simulink model "hand_simulator_v4"  (R2023b)
settings: Solver=VariableStepAuto  StartTime=0.0  StopTime=0  FixedStep=1e-2  RelTol=1e-3
PreLoadFcn:
  | addpath("functions\HandModel\HumanHand\")
undefined symbols (not defined in the file): ts, X, Y, Z
libraries: sm_lib x211, nesl_utility x56
(part 1 of 6)
settings Model: Creator=chopp  LastModifiedBy=chopp
settings ExplorerConfigSet: InternalSimMechanicsExplorerSettings="<ExplorerConfiguration><canonicalview>default</canonicalview><AnimationSetting><BasePlaybackSpeed>1.0</BasePlaybackSpeed><PlaybackSpeedFactor>1.0</PlaybackSpeedFactor></AnimationSetting><TilePanel><TileInfo><Tiles Columns=\"1\" Count=\"1\" Rows=\"1\"><Column Weight=\"1\"/><Row Weight=\"1\"/><Tile Height=\"1\" Width=\"1\" X=\"0\" Y=\"0\"/></Tiles></TileInfo><SceneInfo><SceneViewer><BGColor><R>1</R><G>1</G><B>1</B></BGColor><Camera><DoPerspective>on</DoPerspective><Position><X>0.119329689227050506</X><Y>0.117433489686037784</Y><Z>0.124504754223393604</Z></Position><Center><X>0.0300118695298526722</X><Y>0.0234238145278355299</Y><Z>0.0378621546990252772</Z></Center><Up><X>0.816868216190496765</X><Y>-0.362790797954974598</Y><Z>-0.448451953164381412</Z></Up><ViewLimDist>1</ViewLimDist><YLim>0.466307658154998583</YLim><XLim>0.634472152198297223</XLim></Camera></SceneViewer></SceneInfo></TilePanel><MechEditorPanel><Cameras><Camera><Id>Camera1</Id><Value><Name>Camera1</Name><NativeCamera><PositionKeyframeSet><Keyframe><Time>0</Time><Value><X>0.11932968922705051</X><Y>0.11743348968603778</Y><Z>0.1245047542233936</Z></Value></Keyframe></PositionKeyframeSet><CenterKeyframeSet><Keyframe><Time>0</Time><Value><X>0.030011869529852672</X><Y>0.02342381452783553</Y><Z>0.037862154699025277</Z></Value></Keyframe></CenterKeyframeSet><UpVectorKeyframeSet><Keyframe><Time>0</Time><Value><X>0.81686821619049677</X><Y>-0.3627907979549746</Y><Z>-0.44845195316438141</Z></Value></Keyframe></UpVectorKeyframeSet></NativeCamera></Value></Camera></Cameras><GfxPanelCameraMap><MapElement CameraMLId=\"Camera1\" GfxPanelIndex=\"0\"/></GfxPanelCameraMap><VideoCreator><PlaybackSpeedRatio>1.0</PlaybackSpeedRatio><FrameRate>30</FrameRate><VideoFormat>Motion JPEG AVI</VideoFormat><FrameSize>auto</FrameSize></VideoCreator></MechEditorPanel></ExplorerConfiguration>"

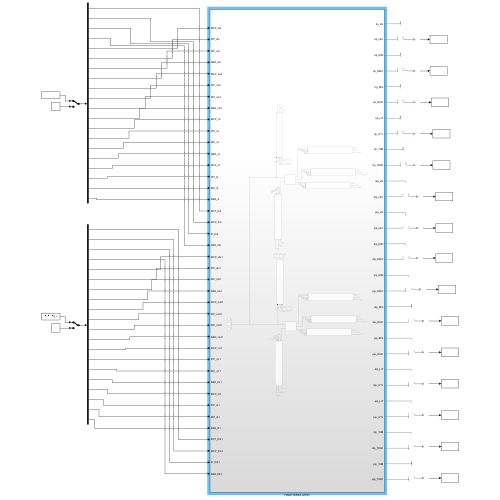
[thumbnail: Simulink's stored preview of the top-level diagram]
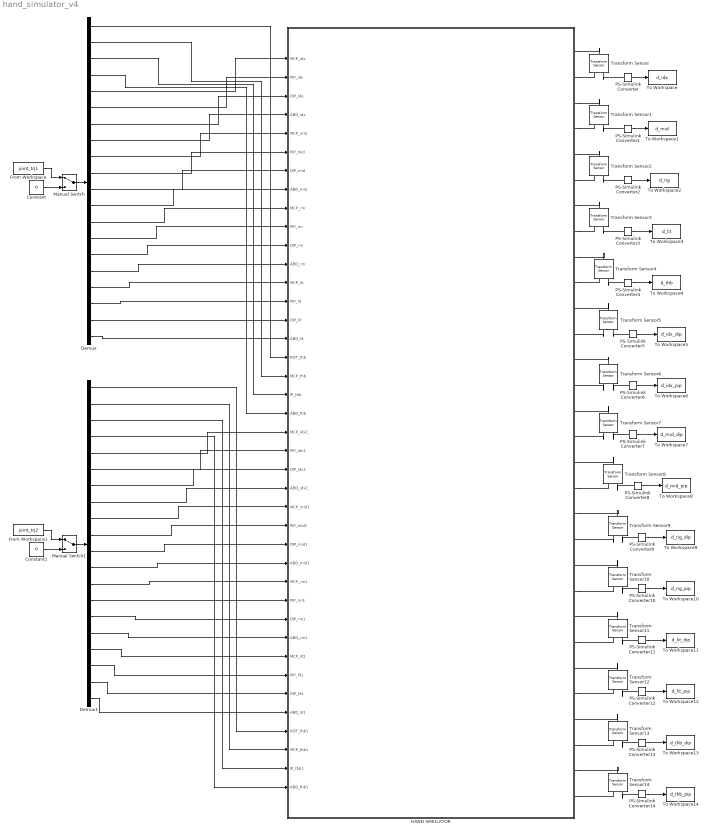
== system hand_simulator_v4 ==
  Constant : Constant  Value=0
  Constant1 : Constant  Value=0
  Demux : Demux  Outputs=20
  Demux1 : Demux  Outputs=20
  From Workspace : FromWorkspace  VariableName=joint_trj1  SampleTime=ts
  From Workspace1 : FromWorkspace  VariableName=joint_trj2  SampleTime=ts
  HAND SIMULATOR : Subsystem
  Manual Switch : ManualSwitch
  Manual Switch1 : ManualSwitch
  PS-Simulink Converter{,1..14} (15 alike) : nesl_utility/PS-Simulink Converter  PhysicalDomain=network_engine_domain  SubClassName=ps_output  LeftPortType=input  RightPortType=output  PseudoPeriodic=off  Frequencies=[]  VectorFormat=inherit  Unit=m  AffineConversion=off
  To Workspace : ToWorkspace  VariableName=d_idx  SaveFormat=Timeseries  SampleTime=0.01
  To Workspace1 : ToWorkspace  VariableName=d_mid  SaveFormat=Timeseries  SampleTime=0.01
  To Workspace10 : ToWorkspace  VariableName=d_rig_pip  SaveFormat=Timeseries  SampleTime=0.01
  To Workspace11 : ToWorkspace  VariableName=d_lit_dip  SaveFormat=Timeseries  SampleTime=0.01
  To Workspace12 : ToWorkspace  VariableName=d_lit_pip  SaveFormat=Timeseries  SampleTime=0.01
  To Workspace13 : ToWorkspace  VariableName=d_thb_dip  SaveFormat=Timeseries  SampleTime=0.01
  To Workspace14 : ToWorkspace  VariableName=d_thb_pip  SaveFormat=Timeseries  SampleTime=0.01
  To Workspace2 : ToWorkspace  VariableName=d_rig  SaveFormat=Timeseries  SampleTime=0.01
  To Workspace3 : ToWorkspace  VariableName=d_lit  SaveFormat=Timeseries  SampleTime=0.01
  To Workspace4 : ToWorkspace  VariableName=d_thb  SaveFormat=Timeseries  SampleTime=0.01
  To Workspace5 : ToWorkspace  VariableName=d_idx_dip  SaveFormat=Timeseries  SampleTime=0.01
  To Workspace6 : ToWorkspace  VariableName=d_idx_pip  SaveFormat=Timeseries  SampleTime=0.01
  To Workspace7 : ToWorkspace  VariableName=d_mid_dip  SaveFormat=Timeseries  SampleTime=0.01
  To Workspace8 : ToWorkspace  VariableName=d_mid_pip  SaveFormat=Timeseries  SampleTime=0.01
  To Workspace9 : ToWorkspace  VariableName=d_rig_dip  SaveFormat=Timeseries  SampleTime=0.01
  Transform Sensor{,1..14} (15 alike) : sm_lib/Frames and Transforms/Transform Sensor  MeasurementFrame=World  RotationSequence=XYX  SenseAngle=off  SenseAxis=off  SenseQ=off  SenseR=off  SenseRotationSequence=off  SenseOmegaX=off  SenseOmegaY=off  SenseOmegaZ=off  SenseOmega=off  SenseQDot=off  SenseRDot=off  SenseRotationSequenceDot=off  SenseAlphaX=off  SenseAlphaY=off  SenseAlphaZ=off  SenseAlpha=off  SenseQDDot=off  SenseRDDot=off  SenseX=off  SenseY=off  SenseZ=off  SenseXYZ=off  SenseRad=off  SenseAzim=off  SenseDist=on  SenseInc=off  SenseXDot=off  SenseYDot=off  SenseZDot=off  SenseXYZDot=off  SenseRadDot=off  SenseAzimDot=off  SenseDistDot=off  SenseIncDot=off  SenseXDDot=off  SenseYDDot=off  SenseZDDot=off  SenseXYZDDot=off  SenseRadDDot=off  SenseAzimDDot=off  SenseDistDDot=off  SenseIncDDot=off
  wires:
  Manual Switch1/1 -> Demux1/1
  Demux1/20 -> HAND SIMULATOR/36(ABD_lit1)
  Manual Switch/1 -> Demux/1
  Demux1/12 -> HAND SIMULATOR/28(ABD_mid1)
  From Workspace/1 -> Manual Switch/1
  Demux/14 -> HAND SIMULATOR/10(PIP_rin)
  Demux/2 -> HAND SIMULATOR/18(MCP_thb)
  Demux1/2 -> HAND SIMULATOR/38(MCP_thb1)
  Demux/17 -> HAND SIMULATOR/13(MCP_lit)
  Constant1/1 -> Manual Switch1/2
  Constant/1 -> Manual Switch/2
  Demux/1 -> HAND SIMULATOR/17(ROT_thb)
  From Workspace1/1 -> Manual Switch1/1
  Demux/18 -> HAND SIMULATOR/14(PIP_lit)
  Demux/3 -> HAND SIMULATOR/19(IP_thb)
  Demux/4 -> HAND SIMULATOR/20(ABD_thb)
  PS-Simulink Converter1/1 -> To Workspace1/1
  Demux/5 -> HAND SIMULATOR/1(MCP_idx)
  Demux/16 -> HAND SIMULATOR/12(ABD_rin)
  Demux/6 -> HAND SIMULATOR/2(PIP_idx)
  Demux/7 -> HAND SIMULATOR/3(DIP_idx)
  Demux/8 -> HAND SIMULATOR/4(ABD_idx)
  Demux/9 -> HAND SIMULATOR/5(MCP_mid)
  Demux/20 -> HAND SIMULATOR/16(ABD_lit)
  Demux/10 -> HAND SIMULATOR/6(PIP_mid)
  Demux/11 -> HAND SIMULATOR/7(DIP_mid)
  Demux/12 -> HAND SIMULATOR/8(ABD_mid)
  Demux/13 -> HAND SIMULATOR/9(MCP_rin)
  Demux/15 -> HAND SIMULATOR/11(DIP_rin)
  Demux1/17 -> HAND SIMULATOR/33(MCP_lit1)
  Demux/19 -> HAND SIMULATOR/15(DIP_lit)
  Demux1/4 -> HAND SIMULATOR/40(ABD_thb1)
  Demux1/1 -> HAND SIMULATOR/37(ROT_thb1)
  Demux1/19 -> HAND SIMULATOR/35(DIP_lit1)
  Demux1/8 -> HAND SIMULATOR/24(ABD_idx1)
  Demux1/3 -> HAND SIMULATOR/39(IP_thb1)
  Demux1/5 -> HAND SIMULATOR/21(MCP_idx1)
  Demux1/6 -> HAND SIMULATOR/22(PIP_idx1)
  Demux1/7 -> HAND SIMULATOR/23(DIP_idx1)
  Demux1/9 -> HAND SIMULATOR/25(MCP_mid1)
  Demux1/10 -> HAND SIMULATOR/26(PIP_mid1)
  Demux1/11 -> HAND SIMULATOR/27(DIP_mid1)
  Demux1/13 -> HAND SIMULATOR/29(MCP_rin1)
  Demux1/14 -> HAND SIMULATOR/30(PIP_rin1)
  Demux1/15 -> HAND SIMULATOR/31(DIP_rin1)
  Demux1/16 -> HAND SIMULATOR/32(ABD_rin1)
  Demux1/18 -> HAND SIMULATOR/34(PIP_lit1)
  PS-Simulink Converter/1 -> To Workspace/1
  PS-Simulink Converter2/1 -> To Workspace2/1
  PS-Simulink Converter3/1 -> To Workspace3/1
  PS-Simulink Converter4/1 -> To Workspace4/1
  PS-Simulink Converter5/1 -> To Workspace5/1
  PS-Simulink Converter6/1 -> To Workspace6/1
  PS-Simulink Converter7/1 -> To Workspace7/1
  PS-Simulink Converter8/1 -> To Workspace8/1
  PS-Simulink Converter9/1 -> To Workspace9/1
  PS-Simulink Converter10/1 -> To Workspace10/1
  PS-Simulink Converter11/1 -> To Workspace11/1
  PS-Simulink Converter12/1 -> To Workspace12/1
  PS-Simulink Converter13/1 -> To Workspace13/1
  PS-Simulink Converter14/1 -> To Workspace14/1
  connections:
  Transform Sensor3/RConn2 -- PS-Simulink Converter3/LConn1
  HAND SIMULATOR/RConn5 -- Transform Sensor2/LConn1
  HAND SIMULATOR/RConn8 -- Transform Sensor3/RConn1
  HAND SIMULATOR/RConn9 -- Transform Sensor4/LConn1
  Transform Sensor1/RConn2 -- PS-Simulink Converter1/LConn1
  Transform Sensor2/RConn2 -- PS-Simulink Converter2/LConn1
  HAND SIMULATOR/RConn3 -- Transform Sensor1/LConn1
  Transform Sensor4/RConn2 -- PS-Simulink Converter4/LConn1
  HAND SIMULATOR/RConn6 -- Transform Sensor2/RConn1
  HAND SIMULATOR/RConn7 -- Transform Sensor3/LConn1
  HAND SIMULATOR/RConn1 -- Transform Sensor/LConn1
  HAND SIMULATOR/RConn2 -- Transform Sensor/RConn1
  HAND SIMULATOR/RConn4 -- Transform Sensor1/RConn1
  HAND SIMULATOR/RConn10 -- Transform Sensor4/RConn1
  Transform Sensor/RConn2 -- PS-Simulink Converter/LConn1
  Transform Sensor5/RConn1 -- HAND SIMULATOR/RConn12
  Transform Sensor5/RConn2 -- PS-Simulink Converter5/LConn1
  Transform Sensor5/LConn1 -- HAND SIMULATOR/RConn11
  Transform Sensor6/RConn2 -- PS-Simulink Converter6/LConn1
  Transform Sensor6/LConn1 -- HAND SIMULATOR/RConn13
  Transform Sensor6/RConn1 -- HAND SIMULATOR/RConn14
  Transform Sensor7/RConn1 -- HAND SIMULATOR/RConn16
  Transform Sensor7/LConn1 -- HAND SIMULATOR/RConn15
  Transform Sensor7/RConn2 -- PS-Simulink Converter7/LConn1
  Transform Sensor8/RConn2 -- PS-Simulink Converter8/LConn1
  HAND SIMULATOR/RConn18 -- Transform Sensor8/RConn1
  Transform Sensor8/LConn1 -- HAND SIMULATOR/RConn17
  Transform Sensor9/RConn2 -- PS-Simulink Converter9/LConn1
  Transform Sensor9/RConn1 -- HAND SIMULATOR/RConn20
  HAND SIMULATOR/RConn19 -- Transform Sensor9/LConn1
  Transform Sensor10/RConn2 -- PS-Simulink Converter10/LConn1
  HAND SIMULATOR/RConn22 -- Transform Sensor10/RConn1
  Transform Sensor10/LConn1 -- HAND SIMULATOR/RConn21
  Transform Sensor11/RConn2 -- PS-Simulink Converter11/LConn1
  HAND SIMULATOR/RConn24 -- Transform Sensor11/RConn1
  Transform Sensor11/LConn1 -- HAND SIMULATOR/RConn23
  Transform Sensor12/RConn2 -- PS-Simulink Converter12/LConn1
  HAND SIMULATOR/RConn26 -- Transform Sensor12/RConn1
  Transform Sensor12/LConn1 -- HAND SIMULATOR/RConn25
  Transform Sensor13/RConn2 -- PS-Simulink Converter13/LConn1
  HAND SIMULATOR/RConn28 -- Transform Sensor13/RConn1
  Transform Sensor13/LConn1 -- HAND SIMULATOR/RConn27
  Transform Sensor14/RConn2 -- PS-Simulink Converter14/LConn1
  HAND SIMULATOR/RConn30 -- Transform Sensor14/RConn1
  HAND SIMULATOR/RConn29 -- Transform Sensor14/LConn1

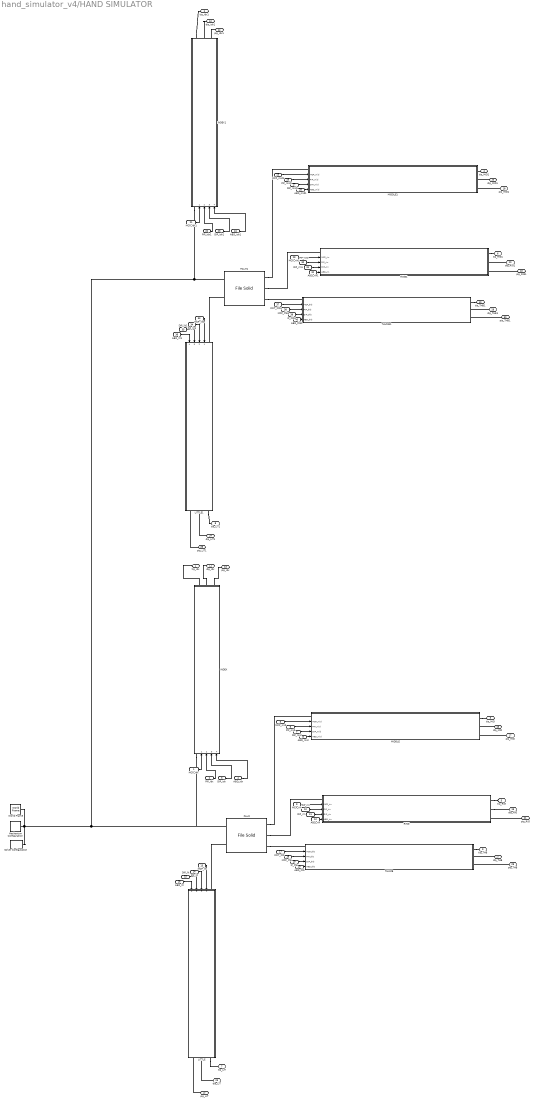
== system hand_simulator_v4/HAND SIMULATOR ==
  MCP_idx : Inport
  PIP_idx : Inport  Port=2
  DIP_idx : Inport  Port=3
  ABD_idx : Inport  Port=4
  MCP_mid : Inport  Port=5
  PIP_mid : Inport  Port=6
  DIP_mid : Inport  Port=7
  ABD_mid : Inport  Port=8
  MCP_rin : Inport  Port=9
  PIP_rin : Inport  Port=10
  DIP_rin : Inport  Port=11
  ABD_rin : Inport  Port=12
  MCP_lit : Inport  Port=13
  PIP_lit : Inport  Port=14
  DIP_lit : Inport  Port=15
  ABD_lit : Inport  Port=16
  ROT_thb : Inport  Port=17
  MCP_thb : Inport  Port=18
  IP_thb : Inport  Port=19
  ABD_thb : Inport  Port=20
  MCP_idx1 : Inport  Port=21
  PIP_idx1 : Inport  Port=22
  DIP_idx1 : Inport  Port=23
  ABD_idx1 : Inport  Port=24
  MCP_mid1 : Inport  Port=25
  PIP_mid1 : Inport  Port=26
  DIP_mid1 : Inport  Port=27
  ABD_mid1 : Inport  Port=28
  MCP_rin1 : Inport  Port=29
  PIP_rin1 : Inport  Port=30
  DIP_rin1 : Inport  Port=31
  ABD_rin1 : Inport  Port=32
  MCP_lit1 : Inport  Port=33
  PIP_lit1 : Inport  Port=34
  DIP_lit1 : Inport  Port=35
  ABD_lit1 : Inport  Port=36
  ROT_thb1 : Inport  Port=37
  MCP_thb1 : Inport  Port=38
  IP_thb1 : Inport  Port=39
  ABD_thb1 : Inport  Port=40
  INDEX : Subsystem
      settings: PortSchema="{\"entries\":[{\"content\":{\"sides\":[{\"content\":{\"connectorIds\":[\"LConn1\",\"In1\",\"In2\",\"In3\",\"In4\"]},\"type\":\"ConnectorPlacement.EquallySpacedRectSide\",\"uuid\":\"ba2071f2-d0ca-4999-8d8c-ca74a0e8f886\"},{\"content\":{\"connectorIds\":[\"RConn1\",\"RConn2\",\"RConn3\"],\"side\":\"RIGHT\"},\"type\":\"ConnectorPlacement.EquallySpacedRectSide\",\"uuid\":\"4961bf0d-9a2d-4923-b4f3-2392b2830b72\"},{\"content\":{\"side\":\"TOP\"},\"type\":\"ConnectorPlacement.EquallySpacedRectSide\",\"uuid\":\"0e6def02-82ab-4410-9cb6-5cc33d72600d\"}]},\"type\":\"ConnectorPlacement.EquallySpacedConnector\",\"uuid\":\"0dbe5955-5a93-4a14-ac05-25d414210df3\"}],\"packageUris\":[\"http://schema.mathworks.com/mf0/Connector/R2020b\"],\"version\":\"1.0\"}"
  INDEX1 : Subsystem
      settings: PortSchema="{\"entries\":[{\"content\":{\"sides\":[{\"content\":{\"connectorIds\":[\"LConn1\",\"In1\",\"In2\",\"In3\",\"In4\"]},\"type\":\"ConnectorPlacement.EquallySpacedRectSide\",\"uuid\":\"ba2071f2-d0ca-4999-8d8c-ca74a0e8f886\"},{\"content\":{\"connectorIds\":[\"RConn1\",\"RConn2\",\"RConn3\"],\"side\":\"RIGHT\"},\"type\":\"ConnectorPlacement.EquallySpacedRectSide\",\"uuid\":\"4961bf0d-9a2d-4923-b4f3-2392b2830b72\"},{\"content\":{\"side\":\"TOP\"},\"type\":\"ConnectorPlacement.EquallySpacedRectSide\",\"uuid\":\"0e6def02-82ab-4410-9cb6-5cc33d72600d\"}]},\"type\":\"ConnectorPlacement.EquallySpacedConnector\",\"uuid\":\"0dbe5955-5a93-4a14-ac05-25d414210df3\"}],\"packageUris\":[\"http://schema.mathworks.com/mf0/Connector/R2020b\"],\"version\":\"1.0\"}"
  LITTLE : Subsystem
      settings: PortSchema="{\"entries\":[{\"content\":{\"sides\":[{\"content\":{\"connectorIds\":[\"LConn1\",\"In1\",\"In2\",\"In3\",\"In4\"]},\"type\":\"ConnectorPlacement.EquallySpacedRectSide\",\"uuid\":\"6da030c9-b445-421e-a3aa-5870985b44ef\"},{\"content\":{\"connectorIds\":[\"RConn1\",\"RConn2\",\"RConn3\"],\"side\":\"RIGHT\"},\"type\":\"ConnectorPlacement.EquallySpacedRectSide\",\"uuid\":\"ddd1b4ad-e82e-4076-8ea7-1e0a4f531141\"},{\"content\":{\"side\":\"TOP\"},\"type\":\"ConnectorPlacement.EquallySpacedRectSide\",\"uuid\":\"430d8793-e7d8-4c1f-b03b-bab4880931cf\"}]},\"type\":\"ConnectorPlacement.EquallySpacedConnector\",\"uuid\":\"9c5926f4-db03-4b4c-81de-0122835d2650\"}],\"packageUris\":[\"http://schema.mathworks.com/mf0/Connector/R2020b\"],\"version\":\"1.0\"}"
  LITTLE1 : Subsystem
      settings: PortSchema="{\"entries\":[{\"content\":{\"sides\":[{\"content\":{\"connectorIds\":[\"LConn1\",\"In1\",\"In2\",\"In3\",\"In4\"]},\"type\":\"ConnectorPlacement.EquallySpacedRectSide\",\"uuid\":\"6da030c9-b445-421e-a3aa-5870985b44ef\"},{\"content\":{\"connectorIds\":[\"RConn1\",\"RConn2\",\"RConn3\"],\"side\":\"RIGHT\"},\"type\":\"ConnectorPlacement.EquallySpacedRectSide\",\"uuid\":\"ddd1b4ad-e82e-4076-8ea7-1e0a4f531141\"},{\"content\":{\"side\":\"TOP\"},\"type\":\"ConnectorPlacement.EquallySpacedRectSide\",\"uuid\":\"430d8793-e7d8-4c1f-b03b-bab4880931cf\"}]},\"type\":\"ConnectorPlacement.EquallySpacedConnector\",\"uuid\":\"9c5926f4-db03-4b4c-81de-0122835d2650\"}],\"packageUris\":[\"http://schema.mathworks.com/mf0/Connector/R2020b\"],\"version\":\"1.0\"}"
  MIDDLE : Subsystem
      settings: PortSchema="{\"entries\":[{\"content\":{\"sides\":[{\"content\":{\"connectorIds\":[\"LConn1\",\"In1\",\"In2\",\"In3\",\"In4\"]},\"type\":\"ConnectorPlacement.EquallySpacedRectSide\",\"uuid\":\"6da030c9-b445-421e-a3aa-5870985b44ef\"},{\"content\":{\"connectorIds\":[\"RConn1\",\"RConn2\",\"RConn3\"],\"side\":\"RIGHT\"},\"type\":\"ConnectorPlacement.EquallySpacedRectSide\",\"uuid\":\"ddd1b4ad-e82e-4076-8ea7-1e0a4f531141\"},{\"content\":{\"side\":\"TOP\"},\"type\":\"ConnectorPlacement.EquallySpacedRectSide\",\"uuid\":\"430d8793-e7d8-4c1f-b03b-bab4880931cf\"}]},\"type\":\"ConnectorPlacement.EquallySpacedConnector\",\"uuid\":\"9c5926f4-db03-4b4c-81de-0122835d2650\"}],\"packageUris\":[\"http://schema.mathworks.com/mf0/Connector/R2020b\"],\"version\":\"1.0\"}"
  MIDDLE1 : Subsystem
      settings: PortSchema="{\"entries\":[{\"content\":{\"sides\":[{\"content\":{\"connectorIds\":[\"LConn1\",\"In1\",\"In2\",\"In3\",\"In4\"]},\"type\":\"ConnectorPlacement.EquallySpacedRectSide\",\"uuid\":\"6da030c9-b445-421e-a3aa-5870985b44ef\"},{\"content\":{\"connectorIds\":[\"RConn1\",\"RConn2\",\"RConn3\"],\"side\":\"RIGHT\"},\"type\":\"ConnectorPlacement.EquallySpacedRectSide\",\"uuid\":\"ddd1b4ad-e82e-4076-8ea7-1e0a4f531141\"},{\"content\":{\"side\":\"TOP\"},\"type\":\"ConnectorPlacement.EquallySpacedRectSide\",\"uuid\":\"430d8793-e7d8-4c1f-b03b-bab4880931cf\"}]},\"type\":\"ConnectorPlacement.EquallySpacedConnector\",\"uuid\":\"9c5926f4-db03-4b4c-81de-0122835d2650\"}],\"packageUris\":[\"http://schema.mathworks.com/mf0/Connector/R2020b\"],\"version\":\"1.0\"}"
  Mechanism Configuration : sm_lib/Utilities/Mechanism Configuration  UniformGravity=Constant  GravityVector=[0 0 0]  GravityVectorUnits=m/s^2  LinearizationDelta=0.001  JointModeTransitionNonlinearIterations=2
  PALM : sm_lib/Body Elements/File Solid  ExtGeomFileName=palm.STEP  UnitType=FromFile  ExtGeomFileUnits=m  StepReaderType=HEX  ExportConvexHullGeometry=off  InertiaType=CalculateFromGeometry  Mass=1  MassUnits=kg  CenterOfMass=[0 0 0]  CenterOfMassUnits=m  MomentsOfInertia=[1 1 1]  MomentsOfInertiaUnits=kg*m^2  ProductsOfInertia=[0 0 0]  ProductsOfInertiaUnits=kg*m^2  BasedOnType=Density  Density=1000  DensityUnits=kg/m^3  DoExposeReferenceFrame=on  SerializedFrames=<Frames><Frame><Id>Frame1</Id><Value><Name>MID</Name><Origin><Source>GeometricFeature</Source><FeatureName>circular curve 11</FeatureName></Origin><PrimaryAxis><DefinedDirection>+Z</DefinedDirection><Source>ReferenceFrame</Source><SourceDirection>+Z</SourceDirection><FeatureName></FeatureName></PrimaryAxis><SecondaryAxis><DefinedDirection>+X</DefinedDirection><Source>ReferenceFrame</Source><SourceDirection>+X</SourceDirection><FeatureName></FeatureName></SecondaryAxis></Value></Frame><Frame><Id>Frame2</Id><Value><Name>RIG</Name><Origin><Source>GeometricFeature</Source><FeatureName>circular curve 6</FeatureName></Origin><PrimaryAxis><DefinedDirection>+Z</DefinedDirection><Source>ReferenceFrame</Source><SourceDirection>+Z</SourceDirection><FeatureName></FeatureName></PrimaryAxis><SecondaryAxis><DefinedDirection>+X</DefinedDirection><Source>ReferenceFrame</Source><SourceDirection>+X</SourceDirection><FeatureName></FeatureName></SecondaryAxis></Value></Frame><Frame><Id>Frame3</Id><Value><Name>LIT</Name><Origin><Source>GeometricFeature</Source><FeatureName>circular curve 2</FeatureName></Origin><PrimaryAxis><DefinedDirection>+Z</DefinedDirection><Source>ReferenceFrame</Source><SourceDirection>+Z</SourceDirection><FeatureName></FeatureName></PrimaryAxis><SecondaryAxis><DefinedDirection>+X</DefinedDirection><Source>ReferenceFrame</Source><SourceDirection>+X</SourceDirection><FeatureName></FeatureName></SecondaryAxis></Value></Frame><Frame><Id>Frame4</Id><Value><Name>THB</Name><Origin><Source>GeometricFeature</Source><FeatureName>circular curve 22</FeatureName></Origin><PrimaryAxis><DefinedDirection>+X</DefinedDirection><Source>ReferenceFrame</Source><SourceDirection>+Z</SourceDirection><FeatureName></FeatureName></PrimaryAxis><SecondaryAxis><DefinedDirection>+Y</DefinedDirection><Source>ReferenceFrame</Source><SourceDirection>+X</SourceDirection><FeatureName></FeatureName></SecondaryAxis></Value></Frame></Frames>  GraphicType=FromGeometry  MarkerShape=Sphere  MarkerSize=10  GraphicVisPropType=SimpleVisualProperties  GraphicDiffuseColor=[0.5 0.5 0.5]  GraphicSpecularColor=[0.5 0.5 0.5 1.0]  GraphicAmbientColor=[0.15 0.15 0.15 1.0]  GraphicEmissiveColor=[0.0 0.0 0.0 1.0]  GraphicShininess=75  GraphicOpacity=1.0
  PALM1 : sm_lib/Body Elements/File Solid  ExtGeomFileName=palm.STEP  UnitType=FromFile  ExtGeomFileUnits=m  StepReaderType=HEX  ExportConvexHullGeometry=off  InertiaType=CalculateFromGeometry  Mass=1  MassUnits=kg  CenterOfMass=[0 0 0]  CenterOfMassUnits=m  MomentsOfInertia=[1 1 1]  MomentsOfInertiaUnits=kg*m^2  ProductsOfInertia=[0 0 0]  ProductsOfInertiaUnits=kg*m^2  BasedOnType=Density  Density=1000  DensityUnits=kg/m^3  DoExposeReferenceFrame=on  SerializedFrames=<Frames><Frame><Id>Frame1</Id><Value><Name>MID</Name><Origin><Source>GeometricFeature</Source><FeatureName>circular curve 11</FeatureName></Origin><PrimaryAxis><DefinedDirection>+Z</DefinedDirection><Source>ReferenceFrame</Source><SourceDirection>+Z</SourceDirection><FeatureName></FeatureName></PrimaryAxis><SecondaryAxis><DefinedDirection>+X</DefinedDirection><Source>ReferenceFrame</Source><SourceDirection>+X</SourceDirection><FeatureName></FeatureName></SecondaryAxis></Value></Frame><Frame><Id>Frame2</Id><Value><Name>RIG</Name><Origin><Source>GeometricFeature</Source><FeatureName>circular curve 6</FeatureName></Origin><PrimaryAxis><DefinedDirection>+Z</DefinedDirection><Source>ReferenceFrame</Source><SourceDirection>+Z</SourceDirection><FeatureName></FeatureName></PrimaryAxis><SecondaryAxis><DefinedDirection>+X</DefinedDirection><Source>ReferenceFrame</Source><SourceDirection>+X</SourceDirection><FeatureName></FeatureName></SecondaryAxis></Value></Frame><Frame><Id>Frame3</Id><Value><Name>LIT</Name><Origin><Source>GeometricFeature</Source><FeatureName>circular curve 2</FeatureName></Origin><PrimaryAxis><DefinedDirection>+Z</DefinedDirection><Source>ReferenceFrame</Source><SourceDirection>+Z</SourceDirection><FeatureName></FeatureName></PrimaryAxis><SecondaryAxis><DefinedDirection>+X</DefinedDirection><Source>ReferenceFrame</Source><SourceDirection>+X</SourceDirection><FeatureName></FeatureName></SecondaryAxis></Value></Frame><Frame><Id>Frame4</Id><Value><Name>THB</Name><Origin><Source>GeometricFeature</Source><FeatureName>circular curve 22</FeatureName></Origin><PrimaryAxis><DefinedDirection>+X</DefinedDirection><Source>ReferenceFrame</Source><SourceDirection>+Z</SourceDirection><FeatureName></FeatureName></PrimaryAxis><SecondaryAxis><DefinedDirection>+Y</DefinedDirection><Source>ReferenceFrame</Source><SourceDirection>+X</SourceDirection><FeatureName></FeatureName></SecondaryAxis></Value></Frame></Frames>  GraphicType=FromGeometry  MarkerShape=Sphere  MarkerSize=10  GraphicVisPropType=SimpleVisualProperties  GraphicDiffuseColor=[1.0 0.0 0.0]  GraphicSpecularColor=[0.5 0.5 0.5 1.0]  GraphicAmbientColor=[0.15 0.15 0.15 1.0]  GraphicEmissiveColor=[0.0 0.0 0.0 1.0]  GraphicShininess=75  GraphicOpacity=1.0
  RING : Subsystem
      settings: PortSchema="{\"entries\":[{\"content\":{\"sides\":[{\"content\":{\"connectorIds\":[\"LConn1\",\"In1\",\"In2\",\"In3\",\"In4\"]},\"type\":\"ConnectorPlacement.EquallySpacedRectSide\",\"uuid\":\"6da030c9-b445-421e-a3aa-5870985b44ef\"},{\"content\":{\"connectorIds\":[\"RConn1\",\"RConn2\",\"RConn3\"],\"side\":\"RIGHT\"},\"type\":\"ConnectorPlacement.EquallySpacedRectSide\",\"uuid\":\"ddd1b4ad-e82e-4076-8ea7-1e0a4f531141\"},{\"content\":{\"side\":\"TOP\"},\"type\":\"ConnectorPlacement.EquallySpacedRectSide\",\"uuid\":\"430d8793-e7d8-4c1f-b03b-bab4880931cf\"}]},\"type\":\"ConnectorPlacement.EquallySpacedConnector\",\"uuid\":\"9c5926f4-db03-4b4c-81de-0122835d2650\"}],\"packageUris\":[\"http://schema.mathworks.com/mf0/Connector/R2020b\"],\"version\":\"1.0\"}"
  RING1 : Subsystem
      settings: PortSchema="{\"entries\":[{\"content\":{\"sides\":[{\"content\":{\"connectorIds\":[\"LConn1\",\"In1\",\"In2\",\"In3\",\"In4\"]},\"type\":\"ConnectorPlacement.EquallySpacedRectSide\",\"uuid\":\"6da030c9-b445-421e-a3aa-5870985b44ef\"},{\"content\":{\"connectorIds\":[\"RConn1\",\"RConn2\",\"RConn3\"],\"side\":\"RIGHT\"},\"type\":\"ConnectorPlacement.EquallySpacedRectSide\",\"uuid\":\"ddd1b4ad-e82e-4076-8ea7-1e0a4f531141\"},{\"content\":{\"side\":\"TOP\"},\"type\":\"ConnectorPlacement.EquallySpacedRectSide\",\"uuid\":\"430d8793-e7d8-4c1f-b03b-bab4880931cf\"}]},\"type\":\"ConnectorPlacement.EquallySpacedConnector\",\"uuid\":\"9c5926f4-db03-4b4c-81de-0122835d2650\"}],\"packageUris\":[\"http://schema.mathworks.com/mf0/Connector/R2020b\"],\"version\":\"1.0\"}"
  Solver Configuration : nesl_utility/Solver Configuration  PhysicalDomain=network_engine_domain  SubClassName=solver  LeftPortType=input  RightPortType=generic  Tones=[]  Harmonics=[]  SimulateNoise=off  Profile=off  UseLocalSampling=off  EnableSwitchedLinearOptims=on  FrequencyDomain=off  UseCCode=off  RelTol=0.001  AbsTol=0.001  MinStep=1e-09  ToWorkspace=off  RevertToSquareIcSolve=off  NumHomotopyIterations=100  PhasorMode=off  PhasorModeNumHarmonics=1  ConsistencySolver=NEWTON_XTOL_AFTER_FTOL  IndexReductionMethod=DerivativeReplacement  DoDC=off  ResidualTolerance=1e-09  ConsistencyTolSource=GLOBAL  ConsistencyAbsTol=0.001  ConsistencyRelTol=0.001  ConsistencyTolFactor=0.001  UseLocalSolver=off  LocalSolverChoice=NE_BACKWARD_EULER_ADVANCER  ResolveIndetEquations=on  FunctionEvalNumThread=1  LocalSolverSampleTime=0.001  DoFixedCost=off  MaxNonlinIter=3  MaxModeIter=2  ComputeImpulses=off  ImpulseIterations=2  LinearAlgebra=auto  LinearAlgebraNumThread=0  EquationFormulation=NE_TIME_EF  DelaysMemoryBudget=1024  AutomaticFiltering=on  FilteringTimeConstant=0.001  PartitionStorageMethod=AS_NEEDED  PartitionMemoryBudget=1024  PartitionMethod=ROBUST  MultibodyUseLocalSolver=off  MultibodyLocalSolverChoice=ODE1  MultibodyLocalSolverSampleTime=0.001
  THUMB : Subsystem
      settings: PortSchema="{\"entries\":[{\"content\":{\"sides\":[{\"content\":{\"connectorIds\":[\"LConn1\",\"In1\",\"In2\",\"In3\",\"In4\"]},\"type\":\"ConnectorPlacement.EquallySpacedRectSide\",\"uuid\":\"ba2071f2-d0ca-4999-8d8c-ca74a0e8f886\"},{\"content\":{\"connectorIds\":[\"RConn1\",\"RConn2\",\"RConn3\"],\"side\":\"RIGHT\"},\"type\":\"ConnectorPlacement.EquallySpacedRectSide\",\"uuid\":\"4961bf0d-9a2d-4923-b4f3-2392b2830b72\"},{\"content\":{\"side\":\"TOP\"},\"type\":\"ConnectorPlacement.EquallySpacedRectSide\",\"uuid\":\"0e6def02-82ab-4410-9cb6-5cc33d72600d\"}]},\"type\":\"ConnectorPlacement.EquallySpacedConnector\",\"uuid\":\"0dbe5955-5a93-4a14-ac05-25d414210df3\"}],\"packageUris\":[\"http://schema.mathworks.com/mf0/Connector/R2020b\"],\"version\":\"1.0\"}"
  THUMB1 : Subsystem
      settings: PortSchema="{\"entries\":[{\"content\":{\"sides\":[{\"content\":{\"connectorIds\":[\"LConn1\",\"In1\",\"In2\",\"In3\",\"In4\"]},\"type\":\"ConnectorPlacement.EquallySpacedRectSide\",\"uuid\":\"ba2071f2-d0ca-4999-8d8c-ca74a0e8f886\"},{\"content\":{\"connectorIds\":[\"RConn1\",\"RConn2\",\"RConn3\"],\"side\":\"RIGHT\"},\"type\":\"ConnectorPlacement.EquallySpacedRectSide\",\"uuid\":\"4961bf0d-9a2d-4923-b4f3-2392b2830b72\"},{\"content\":{\"side\":\"TOP\"},\"type\":\"ConnectorPlacement.EquallySpacedRectSide\",\"uuid\":\"0e6def02-82ab-4410-9cb6-5cc33d72600d\"}]},\"type\":\"ConnectorPlacement.EquallySpacedConnector\",\"uuid\":\"0dbe5955-5a93-4a14-ac05-25d414210df3\"}],\"packageUris\":[\"http://schema.mathworks.com/mf0/Connector/R2020b\"],\"version\":\"1.0\"}"
  World Frame : sm_lib/Frames and Transforms/World Frame
  tip_idx : PMIOPort  Side=Right
  tip_idx1 : PMIOPort  Port=2  Side=Right
  tip_MID : PMIOPort  Port=3  Side=Right
  tip_MID1 : PMIOPort  Port=4  Side=Right
  tip_RIG : PMIOPort  Port=5  Side=Right
  tip_RIG1 : PMIOPort  Port=6  Side=Right
  tip_LIT : PMIOPort  Port=7  Side=Right
  tip_LIT1 : PMIOPort  Port=8  Side=Right
  tip_THB : PMIOPort  Port=9  Side=Right
  tip_THB1 : PMIOPort  Port=10  Side=Right
  dip_idx : PMIOPort  Port=11  Side=Right
  dip_idx1 : PMIOPort  Port=12  Side=Right
  pip_idx : PMIOPort  Port=13  Side=Right
  pip_idx1 : PMIOPort  Port=14  Side=Right
  dip_MID : PMIOPort  Port=15  Side=Right
  dip_MID1 : PMIOPort  Port=16  Side=Right
  pip_MID : PMIOPort  Port=17  Side=Right
  pip_MID1 : PMIOPort  Port=18  Side=Right
  dip_RIG : PMIOPort  Port=19  Side=Right
  dip_RIG1 : PMIOPort  Port=20  Side=Right
  pip_RIG : PMIOPort  Port=21  Side=Right
  pip_RIG1 : PMIOPort  Port=22  Side=Right
  dip_LIT : PMIOPort  Port=23  Side=Right
  dip_LIT1 : PMIOPort  Port=24  Side=Right
  pip_LIT : PMIOPort  Port=25  Side=Right
  pip_LIT1 : PMIOPort  Port=26  Side=Right
  dip_THB : PMIOPort  Port=27  Side=Right
  dip_THB1 : PMIOPort  Port=28  Side=Right
  pip_THB : PMIOPort  Port=29  Side=Right
  pip_THB1 : PMIOPort  Port=30  Side=Right
  wires:
  IP_thb/1 -> THUMB/3(DIP_thb)
  DIP_lit/1 -> LITTLE/3(DIP_lit)
  ABD_mid/1 -> MIDDLE/4(ABD_mid)
  ABD_rin/1 -> RING/4(ABD_rin)
  ABD_idx/1 -> INDEX/4(ABD_idx)
  MCP_lit/1 -> LITTLE/1(MCP_lit)
  DIP_rin/1 -> RING/3(DIP_rin)
  ABD_lit/1 -> LITTLE/4(ABD_lit)
  PIP_idx/1 -> INDEX/2(PIP_idx)
  MCP_mid/1 -> MIDDLE/1(MCP_mid)
  PIP_mid/1 -> MIDDLE/2(PIP_mid)
  DIP_idx/1 -> INDEX/3(DIP_idx)
  MCP_rin/1 -> RING/1(MCP_rin)
  DIP_mid/1 -> MIDDLE/3(DIP_mid)
  ROT_thb/1 -> THUMB/1(MCP_thb)
  PIP_rin/1 -> RING/2(PIP_rin)
  MCP_idx/1 -> INDEX/1(MCP_idx)
  MCP_thb/1 -> THUMB/2(PIP_thb)
  PIP_lit/1 -> LITTLE/2(PIP_lit)
  ABD_thb/1 -> THUMB/4(ABD_thb)
  ABD_thb1/1 -> THUMB1/4(ABD_thb)
  PIP_lit1/1 -> LITTLE1/2(PIP_lit)
  MCP_thb1/1 -> THUMB1/2(PIP_thb)
  MCP_idx1/1 -> INDEX1/1(MCP_idx)
  PIP_rin1/1 -> RING1/2(PIP_rin)
  ROT_thb1/1 -> THUMB1/1(MCP_thb)
  DIP_mid1/1 -> MIDDLE1/3(DIP_mid)
  MCP_rin1/1 -> RING1/1(MCP_rin)
  DIP_idx1/1 -> INDEX1/3(DIP_idx)
  PIP_mid1/1 -> MIDDLE1/2(PIP_mid)
  MCP_mid1/1 -> MIDDLE1/1(MCP_mid)
  PIP_idx1/1 -> INDEX1/2(PIP_idx)
  ABD_lit1/1 -> LITTLE1/4(ABD_lit)
  DIP_rin1/1 -> RING1/3(DIP_rin)
  MCP_lit1/1 -> LITTLE1/1(MCP_lit)
  ABD_idx1/1 -> INDEX1/4(ABD_idx)
  ABD_rin1/1 -> RING1/4(ABD_rin)
  ABD_mid1/1 -> MIDDLE1/4(ABD_mid)
  DIP_lit1/1 -> LITTLE1/3(DIP_lit)
  IP_thb1/1 -> THUMB1/3(DIP_thb)
  connections:
  PALM1/RConn1 -- Solver Configuration/RConn1 -- World Frame/RConn1 -- Mechanism Configuration/RConn1 -- PALM/RConn1 -- INDEX/LConn1 -- INDEX1/LConn1
  PALM/LConn3 -- THUMB/LConn1
  MIDDLE/RConn1 -- tip_MID/RConn1
  INDEX/RConn1 -- tip_idx/RConn1
  PALM/LConn1 -- MIDDLE/LConn1
  PALM/LConn2 -- RING/LConn1
  PALM/RConn2 -- LITTLE/LConn1
  THUMB/RConn1 -- tip_THB/RConn1
  RING/RConn1 -- tip_RIG/RConn1
  LITTLE/RConn1 -- tip_LIT/RConn1
  LITTLE1/RConn1 -- tip_LIT1/RConn1
  RING1/RConn1 -- tip_RIG1/RConn1
  THUMB1/RConn1 -- tip_THB1/RConn1
  PALM1/RConn2 -- LITTLE1/LConn1
  PALM1/LConn1 -- MIDDLE1/LConn1
  MIDDLE1/RConn1 -- tip_MID1/RConn1
  PALM1/LConn2 -- RING1/LConn1
  PALM1/LConn3 -- THUMB1/LConn1
  INDEX1/RConn1 -- tip_idx1/RConn1
  dip_idx/RConn1 -- INDEX/RConn2
  dip_idx1/RConn1 -- INDEX1/RConn2
  INDEX/RConn3 -- pip_idx/RConn1
  pip_idx1/RConn1 -- INDEX1/RConn3
  dip_MID/RConn1 -- MIDDLE/RConn2
  dip_MID1/RConn1 -- MIDDLE1/RConn2
  pip_MID/RConn1 -- MIDDLE/RConn3
  pip_MID1/RConn1 -- MIDDLE1/RConn3
  RING/RConn2 -- dip_RIG/RConn1
  dip_RIG1/RConn1 -- RING1/RConn2
  pip_RIG/RConn1 -- RING/RConn3
  pip_RIG1/RConn1 -- RING1/RConn3
  dip_LIT/RConn1 -- LITTLE/RConn2
  dip_LIT1/RConn1 -- LITTLE1/RConn2
  pip_LIT/RConn1 -- LITTLE/RConn3
  pip_LIT1/RConn1 -- LITTLE1/RConn3
  dip_THB/RConn1 -- THUMB/RConn2
  dip_THB1/RConn1 -- THUMB1/RConn2
  pip_THB/RConn1 -- THUMB/RConn3
  pip_THB1/RConn1 -- THUMB1/RConn3
